simulink library "MOTORS"  (R2024b)
settings: Solver=VariableStepAuto  StartTime=0.0  StopTime=10.0  RelTol=1e-3
libraries: fl_lib x6, nesl_utility x3, ee_lib x1, slpidlib x1
settings Model: Creator=Mohammed Hany  LastModifiedBy=Mohammed Hany

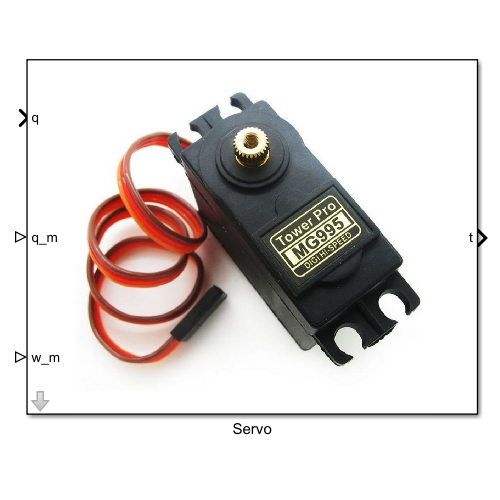
[thumbnail: Simulink's stored preview of the top-level diagram]
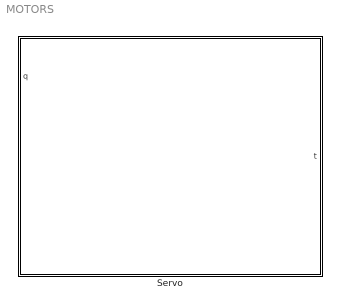
== system MOTORS ==
  Servo : Subsystem  mask{J=0.01, J_unit=cm^2*g, La=12e-6, La_unit=H, P_rated=0.08, P_rated_unit=W, V_i_noload=1.5, V_i_noload_unit=V, V_rated=1.5, V_rated_unit=V, i_noload=0, i_noload_unit=A, w_max=19100, w_max_unit=rpm, w_rated=15000, w_rated_unit=rpm, ratio=5}
      mask prompts: J "physmod:ee:library:comments:electromech:brushed:dc_motor_base:J"; La "physmod:ee:library:comments:electromech:brushed:dc_motor_base:La"; P_rated "physmod:ee:library:comments:electromech:brushed:dc_motor_base:P_rated"; V_i_noload "physmod:ee:library:comments:electromech:brushed:dc_motor_base:V_i_noload"; V_rated "physmod:ee:library:comments:electromech:brushed:dc_motor_base:V_rated"; i_noload "physmod:ee:library:comments:electromech:brushed:dc_motor_base:i_noload"; w_max "physmod:ee:library:comments:electromech:brushed:dc_motor_base:w_max"; w_rated "physmod:ee:library:comments:electromech:brushed:dc_motor_base:w_rated"; ratio "physmod:simscape:library:comments:mechanical:mechanisms:gear_box:ratio"
      mask TypeOptions J: DC Motor/J
      mask TypeOptions J_unit: DC Motor/J_unit
      mask TypeOptions La: DC Motor/La
      mask TypeOptions La_unit: DC Motor/La_unit
      mask TypeOptions P_rated: DC Motor/P_rated
      mask TypeOptions P_rated_unit: DC Motor/P_rated_unit
      mask TypeOptions V_i_noload: DC Motor/V_i_noload
      mask TypeOptions V_i_noload_unit: DC Motor/V_i_noload_unit
      mask TypeOptions V_rated: DC Motor/V_rated
      mask TypeOptions V_rated_unit: DC Motor/V_rated_unit
      mask TypeOptions i_noload: DC Motor/i_noload
      mask TypeOptions i_noload_unit: DC Motor/i_noload_unit
      mask TypeOptions w_max: DC Motor/w_max
      mask TypeOptions w_max_unit: DC Motor/w_max_unit
      mask TypeOptions w_rated: DC Motor/w_rated
      mask TypeOptions w_rated_unit: DC Motor/w_rated_unit
      mask TypeOptions ratio: Gear Box/ratio
      mask DialogControl J Prompt: Rotor inertia
      mask DialogControl La Prompt: Armature inductance
      mask DialogControl P_rated Prompt: Rated load (mechanical power)
      mask DialogControl V_i_noload Prompt: DC supply voltage when measuring no-load current
      mask DialogControl V_rated Prompt: Rated DC supply voltage
      mask DialogControl i_noload Prompt: No-load current
      mask DialogControl w_max Prompt: No-load speed
      mask DialogControl w_rated Prompt: Rated speed (at rated load)
      mask DialogControl ratio Prompt: Gear ratio
      mask Display: image('servo_motor.jpg', [0.5,0.5,0.5,0.5,100,100]);

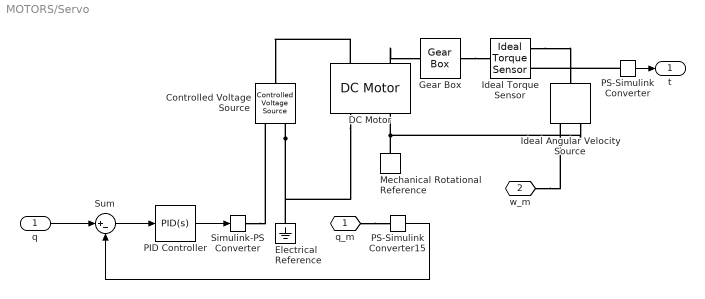
== system MOTORS/Servo ==
  q : Inport
  Controlled Voltage Source : fl_lib/Electrical/Electrical Sources/Controlled Voltage Source
  DC Motor : ee_lib/Electromechanical/Brushed Motors/DC Motor  field_option=ee.enum.field_option.pm  Rf=100 Ohm  Lf=1 H  Laf=0.15 H  If0=0 A  parameterization=ee.enum.dcparam_option.load_speed  Ra=3.9 Ohm  La=La H  emf_or_torque=ee.enum.emf_or_torque.kv  Kv=0.072e-3 V/rpm  Ki=6.876e-4 N*m/A  T_stall=0.24e-3 N*m  w_max=w_max rpm  w_rated=w_rated rpm  P_rated=P_rated W  V_rated=V_rated V  lam_param=ee.enum.lam_param.current  i_noload=i_noload A  V_i_noload=V_i_noload V  J=J cm^2*g  lam=0 N*m*s/rad  speed0=0 rpm  t_fault_armature=1 s  t_fault_field=1 s  fault_action=simscape.enum.assert.action.none  alpha=3.93e-3 1/K  Tmeas=25 degC  thermal_mass=100 J/K  initial_temperature=25 degC
  Electrical Reference : fl_lib/Electrical/Electrical Elements/Electrical Reference
  Gear Box : fl_lib/Mechanical/Mechanisms/Gear Box  ratio=ratio  t_in_specify=off  t_in_priority=None  t_in=0 N*m  t_in_nominal_specify=off  t_in_nominal_value=1  t_in_nominal_unit=N*m  t_out_specify=off  t_out_priority=None  t_out=0 N*m  t_out_nominal_specify=off  t_out_nominal_value=1  t_out_nominal_unit=N*m
  Ideal Angular Velocity Source : fl_lib/Mechanical/Mechanical Sources/Ideal Angular Velocity Source
  Ideal Torque Sensor : fl_lib/Mechanical/Mechanical Sensors/Ideal Torque Sensor
  Mechanical Rotational Reference : fl_lib/Mechanical/Rotational Elements/Mechanical Rotational Reference
  PID Controller : slpidlib/PID Controller  Controller=PID  Form=Parallel  TimeDomain=Continuous-time  UseExternalTs=off  SampleTime=-1  IntegratorMethod=Forward Euler  FilterMethod=Forward Euler  ControllerParametersSource=internal  P=10  I=0  UseKiTs=off  D=0  UseExternalDerivativeSource=off  N=0  UseFilter=on  TunerSelectOption=Transfer Function Based (PID Tuner App)  InitialConditionSource=internal  InitialConditionForIntegrator=0  InitialConditionForFilter=0  DifferentiatorICPrevScaledInput=0  ExternalReset=none  TrackingMode=off  Kt=1  LimitOutput=off  SatLimitsSource=internal  UpperSaturationLimit=inf  LowerSaturationLimit=-inf  LinearizeAsGain=on  AntiWindupMode=none  Kb=1  LimitIntegrator=off  UpperIntegratorSaturationLimit=inf  LowerIntegratorSaturationLimit=-inf  POutMin=[]  POutMax=[]  IOutMin=[]  IOutMax=[]  DOutMin=[]  DOutMax=[]  NOutMin=[]  NOutMax=[]  SumOutMin=[]  SumOutMax=[]  SaturationOutMin=[]  SaturationOutMax=[]  PParamMin=[]  PParamMax=[]  IParamMin=[]  IParamMax=[]  DParamMin=[]  DParamMax=[]  NParamMin=[]  NParamMax=[]  KbParamMin=[]  KbParamMax=[]  KtParamMin=[]  KtParamMax=[]  KbOutMin=[]  KbOutMax=[]  KtOutMin=[]  KtOutMax=[]  IntegratorOutMin=[]  IntegratorOutMax=[]  FilterOutMin=[]  FilterOutMax=[]  SumI1OutMin=[]  SumI1OutMax=[]  SumI2OutMin=[]  SumI2OutMax=[]  SumI3OutMin=[]  SumI3OutMax=[]  SumI4OutMin=[]  SumI4OutMax=[]  SumDOutMin=[]  SumDOutMax=[]  DifferentiatorOutMin=[]  DifferentiatorOutMax=[]  FilterDiffOutCoefMin=[]  FilterDiffOutCoefMax=[]  ReciprocalOutMin=[]  ReciprocalOutMax=[]  SumDenOutMin=[]  SumDenOutMax=[]  SumNumOutMin=[]  SumNumOutMax=[]  DivideOutMin=[]  DivideOutMax=[]  UdiffTsProdOutMin=[]  UdiffTsProdOutMax=[]  NTsProdOutMin=[]  NTsProdOutMax=[]  UintegralTsProdOutMin=[]  UintegralTsProdOutMax=[]  UngainTsProdOutMin=[]  UngainTsProdOutMax=[]  ClampingZeroOutDataTypeStr=Inherit: Inherit via back propagation  ClampingZeroOutMin=[]  ClampingZeroOutMax=[]  FilterDenConstantOutDataTypeStr=Inherit: Inherit via back propagation  FilterDenConstantOutMin=[]  FilterDenConstantOutMax=[]  PCopyOutDataTypeStr=Inherit: Inherit via back propagation  PCopyOutMin=[]  PCopyOutMax=[]  NCopyOutDataTypeStr=Inherit: Inherit via back propagation  NCopyOutMin=[]  NCopyOutMax=[]  IntegratorContinuousStateAttributes=''  IntegratorStateMustResolveToSignalObject=off  IntegratorRTWStateStorageClass=Auto  FilterContinuousStateAttributes=''  FilterStateMustResolveToSignalObject=off  FilterRTWStateStorageClass=Auto  ParallelPVariant=InternalParameters  IdealPVariant=Disabled  IVariant=InternalParameters  DVariant=InternalParameters  IntegratorVariant=Continuous  SatVariant=Disabled  AWVariant=Passthrough  PCopyVariant=Disabled  TRVariant=Disabled  FdbkBlocksVariant=Forward  IdealPFdbkVariant=Disabled  SatFdbkVariant=Disabled  DerivativeFilterVariant=ContFilter  NVariant=InternalParameters  NCopyVariant=Disabled  FilterICVariant=InternalICsFilter  IntegratorICVariant=InternalICs  ExternalResetVariant=Disabled  TRSumVariant=Passthrough  SumFdbkVariant=Disabled  SumVariant=Sum_PID  TsampFilterVariant=InternalTs  TsampNgainVariant=Passthrough  TsampIntegralVariant=Disabled_SignalSpec  ExternalSaturationOutDataTypeStr=Inherit: Same as second input  DerivativeSourceVariant=ErrorSignal  PreIntVariant=InternalPreInt
  PS-Simulink Converter : nesl_utility/PS-Simulink Converter  PhysicalDomain=network_engine_domain  SubClassName=ps_output  LeftPortType=input  RightPortType=output  PseudoPeriodic=off  Frequencies=[]  VectorFormat=inherit  Unit=N*mm  AffineConversion=off
  PS-Simulink Converter15 : nesl_utility/PS-Simulink Converter  PhysicalDomain=network_engine_domain  SubClassName=ps_output  LeftPortType=input  RightPortType=output  PseudoPeriodic=off  Frequencies=[]  VectorFormat=inherit  Unit=deg  AffineConversion=off
  Simulink-PS Converter : nesl_utility/Simulink-PS Converter  PhysicalDomain=network_engine_domain  SubClassName=ps_input  LeftPortType=input  RightPortType=output  PseudoPeriodic=off  Frequencies=[]  NoiseDistribution=none  NoiseParameters=[]  Unit=1  AffineConversion=off  FilteringAndDerivatives=provide  SimscapeFilterOrder=1  InputFilterTimeConstant=0.001  UdotUserProvided=0
  Sum : Sum  Inputs=|+-
  q_m : PMIOPort  Side=Left
  w_m : PMIOPort  Port=2  Side=Left
  t : Outport
  wires:
  PID Controller/1 -> Simulink-PS Converter/1
  PS-Simulink Converter/1 -> t/1
  q/1 -> Sum/1
  PS-Simulink Converter15/1 -> Sum/2
  Sum/1 -> PID Controller/1
  connections:
  Ideal Torque Sensor/RConn1 -- Ideal Angular Velocity Source/LConn1
  Ideal Angular Velocity Source/RConn2 -- DC Motor/RConn2 -- Mechanical Rotational Reference/LConn1
  Controlled Voltage Source/RConn2 -- Electrical Reference/LConn1 -- DC Motor/RConn1
  DC Motor/LConn2 -- Gear Box/LConn1
  PS-Simulink Converter/LConn1 -- Ideal Torque Sensor/RConn2
  DC Motor/LConn1 -- Controlled Voltage Source/LConn1
  Gear Box/RConn1 -- Ideal Torque Sensor/LConn1
  Simulink-PS Converter/RConn1 -- Controlled Voltage Source/RConn1
  w_m/RConn1 -- Ideal Angular Velocity Source/RConn1
  q_m/RConn1 -- PS-Simulink Converter15/LConn1
